simulink model "untitled"  (R2020b)
settings: Solver=VariableStepAuto  StartTime=0.0  StopTime=20  RelTol=1e-3
libraries: simulink x20
settings Model: Creator=pellizzar1  LastModifiedBy=pellizzar1

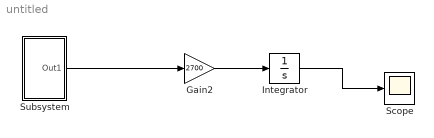
== system untitled ==
  Gain2 : Gain  Gain=2700
  Integrator : Integrator
  Scope : Scope
  Subsystem : Subsystem
  wires:
  Integrator/1 -> Scope/1
  Gain2/1 -> Integrator/1
  Subsystem/1(Out1) -> Gain2/1

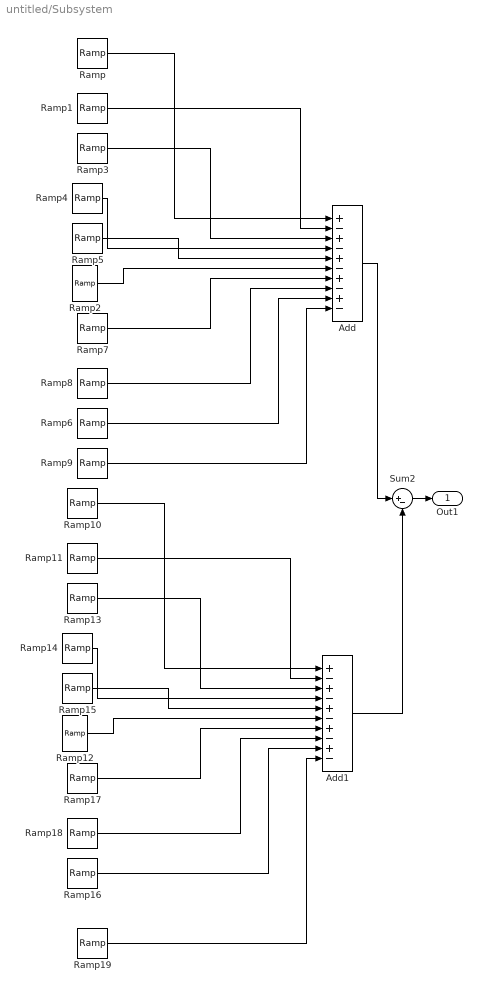
== system untitled/Subsystem ==
  Add : Sum  Inputs=+-+-+-+-+-
  Add1 : Sum  Inputs=+-+-+-+-+-
  Ramp : simulink/Sources/Ramp  slope=1  start=0  InitialOutput=0
  Ramp1 : simulink/Sources/Ramp  slope=2  start=1  InitialOutput=0
  Ramp10 : simulink/Sources/Ramp  slope=2  start=10  InitialOutput=0
  Ramp11 : simulink/Sources/Ramp  slope=2  start=11  InitialOutput=0
  Ramp12 : simulink/Sources/Ramp  slope=2  start=15  InitialOutput=0
  Ramp13 : simulink/Sources/Ramp  slope=2  start=12  InitialOutput=0
  Ramp14 : simulink/Sources/Ramp  slope=2  start=13  InitialOutput=0
  Ramp15 : simulink/Sources/Ramp  slope=2  start=14  InitialOutput=0
  Ramp16 : simulink/Sources/Ramp  slope=2  start=18  InitialOutput=0
  Ramp17 : simulink/Sources/Ramp  slope=2  start=16  InitialOutput=0
  Ramp18 : simulink/Sources/Ramp  slope=2  start=17  InitialOutput=0
  Ramp19 : simulink/Sources/Ramp  slope=1  start=19  InitialOutput=0
  Ramp2 : simulink/Sources/Ramp  slope=2  start=5  InitialOutput=0
  Ramp3 : simulink/Sources/Ramp  slope=2  start=2  InitialOutput=0
  Ramp4 : simulink/Sources/Ramp  slope=2  start=3  InitialOutput=0
  Ramp5 : simulink/Sources/Ramp  slope=2  start=4  InitialOutput=0
  Ramp6 : simulink/Sources/Ramp  slope=2  start=8  InitialOutput=0
  Ramp7 : simulink/Sources/Ramp  slope=2  start=6  InitialOutput=0
  Ramp8 : simulink/Sources/Ramp  slope=2  start=7  InitialOutput=0
  Ramp9 : simulink/Sources/Ramp  slope=1  start=9  InitialOutput=0
  Sum2 : Sum  Inputs=|+-
  Out1 : Outport
  wires:
  Add/1 -> Sum2/1
  Sum2/1 -> Out1/1
  Ramp11/1 -> Add1/2
  Ramp17/1 -> Add1/7
  Ramp13/1 -> Add1/3
  Ramp18/1 -> Add1/8
  Ramp12/1 -> Add1/6
  Ramp14/1 -> Add1/4
  Ramp10/1 -> Add1/1
  Ramp2/1 -> Add/6
  Ramp19/1 -> Add1/10
  Ramp15/1 -> Add1/5
  Ramp16/1 -> Add1/9
  Ramp5/1 -> Add/5
  Ramp3/1 -> Add/3
  Ramp1/1 -> Add/2
  Ramp6/1 -> Add/9
  Add1/1 -> Sum2/2
  Ramp/1 -> Add/1
  Ramp8/1 -> Add/8
  Ramp9/1 -> Add/10
  Ramp4/1 -> Add/4
  Ramp7/1 -> Add/7
